simulink model "neoArm_14_05_2024"  (R2023a)
settings: Solver=VariableStepAuto  StartTime=0.0  StopTime=16  FixedStep=0.001  RelTol=1e-3
values from neighbouring files (symbols this model uses):
  dq0 = [0;0;0;0;0]    [neoArm_main.m]
  K = [1000  900]    [neoArm_main.m]
  objectPos = 0.2    [neoArm_main.m]
  orientations = pi/2*[ones(length(temp1),1) zeros(length(temp1),1) zeros(length(temp1),1)]'    [nesneTakip.m]
  q0 = [0;0;0;0;0]    [neoArm_main.m]
  q1 = [pi/2;0;0;0;0]    [neoArm_main.m]
  refPos = 0.0    (= 0)    [neoArm_main.m]
  tDuration = 16    [neoArm_main.m]
  temp3_x = temp3(1,:)    [nokta_duzenle.m]
  temp3_y = temp3(2,:)    [nokta_duzenle.m]
  temp3_z = temp3(3,:)    [nokta_duzenle.m]
  ts = 0.02    [neoArm_main.m]
  tStart = 0.05    [neoArm_main.m]
  waypoints = temp1'    [nesneTakip.m]
  waypointTimes = linspace(0,tDuration,sayi)    [neoArm_main.m]
  weights = [0 0 0 1 1 1]    [neoArm_main.m]
  wp_js_time = [0 0.001 0.002 0.003 0.004 0.005 0.006 0.007 0.008 0.009 0.01 0.011 ... (16001 elements, 16001x1)]    [joint_space_waypoints.mat]    (also in nokta_duzenle.m = wp_joint_space.Time)
undefined symbols (not defined in the file or in its folder): eul2tform, Levenberg, Marquardt, trvec2tform, X, Y, Z
libraries: sm_lib x69, nesl_utility x37, robotcorelib x10, robotmaniplib x9, simulink x2
(part 1 of 3)
settings Model: SimulationMode=accelerator  PacingRate=0.110000  Creator=guven  LastModifiedBy=guven
settings SolverCC: ZeroCrossAlgorithm=Adaptive
settings DataIOCC: ReturnWorkspaceOutputs=off
settings DebuggingCC: IgnoredZcDiagnostic=none
settings ModelReferenceCC: EnableRefExpFcnMdlSchedulingChecks=on

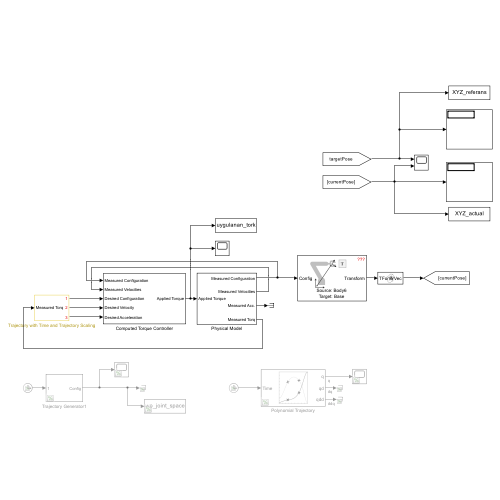
[thumbnail: Simulink's stored preview of the top-level diagram]
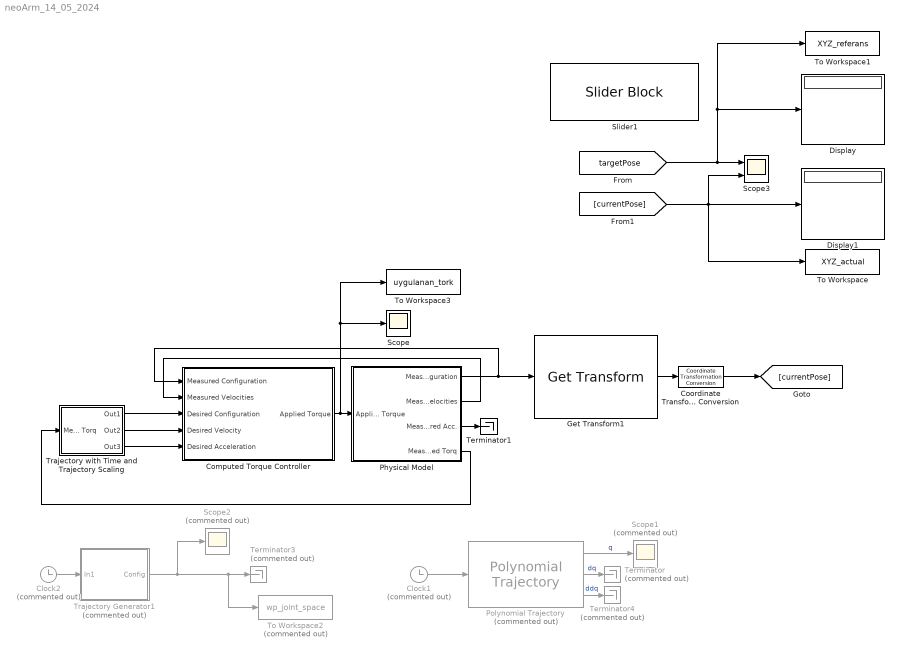
== system neoArm_14_05_2024 ==
  Clock1 : Clock  Commented=on
  Clock2 : Clock  Commented=on
  Computed Torque Controller : Subsystem
  Coordinate Transformation Conversion : robotcorelib/Coordinate Transformation Conversion  InputRepresentation=Homogeneous Transformation  InputEulerSequence=ZYX  ShowTrVecInputPort=on  OutputRepresentation=Translation Vector  OutputEulerSequence=ZYX  ShowTrVecOutputPort=on  SimulateUsing=Interpreted execution
      settings: LibrarySourceBlock=navlib/Utilities/Coordinate Transformation Conversion
  Display : Display
  Display1 : Display
  Get Transform1 : robotmaniplib/Get Transform  RigidBodyTree=neoArm  SourceBody=Body6  TargetBody=Base  SimulateUsing=Interpreted execution
  Physical Model : Subsystem
  Polynomial Trajectory : robotcorelib/Polynomial Trajectory  Commented=on  WaypointSource=Internal  Waypoints=wp_js'  TimePoints=wp_js_time'  TimeInterval=[ 1, 4 ]  Method=Quintic Polynomial  ParameterSource=Internal  VelocityBoundaryCondition=zeros(numel(wp_js_time),5)'  AccelerationBoundaryCondition=zeros(numel(wp_js_time),5)'  SimulateUsing=Interpreted execution
  Scope : Scope
  Scope1 : Scope  Commented=on
  Scope2 : Scope  Commented=on
  Scope3 : Scope  NumInputPorts=2
  Slider1 : SliderBlock  ScaleMin=0.0  ScaleMax=1
  Terminator : Terminator  Commented=on
  Terminator1 : Terminator
  Terminator3 : Terminator  Commented=on
  Terminator4 : Terminator  Commented=on
  To Workspace : ToWorkspace  VariableName=XYZ_actual  SaveFormat=Timeseries  SampleTime=-1
  To Workspace1 : ToWorkspace  VariableName=XYZ_referans  SaveFormat=Timeseries  SampleTime=-1
  To Workspace2 : ToWorkspace  Commented=on  VariableName=wp_joint_space  SaveFormat=Timeseries  SampleTime=-1
  To Workspace3 : ToWorkspace  VariableName=uygulanan_tork  SampleTime=-1
  Trajectory Generator1 : Subsystem  Commented=on
  Trajectory with Time and Trajectory Scaling : Subsystem
  wires:
  Physical Model/2(Measured Velocities) -> Computed Torque Controller/2(Measured Velocities)
  Physical Model/3(Measured Acc.) -> Terminator1/1
  Computed Torque Controller/1(Applied Torque) -> To Workspace3/1, Scope/1, Physical Model/1(Applied Torque)
  [targetPose] -> Display/1, To Workspace1/1, Scope3/1
  [currentPose] -> To Workspace/1, Display1/1, Scope3/2
  Physical Model/4(Measured Torq) -> Trajectory with Time and Trajectory Scaling/1(Measured Torq)
  Trajectory with Time and Trajectory Scaling/1(Out1) -> Computed Torque Controller/3(Desired Configuration)
  Trajectory with Time and Trajectory Scaling/2(Out2) -> Computed Torque Controller/4(Desired Velocity)
  Trajectory with Time and Trajectory Scaling/3(Out3) -> Computed Torque Controller/5(Desired Acceleration)
  Physical Model/1(Measured Configuration) -> Get Transform1/1, Computed Torque Controller/1(Measured Configuration)
  Coordinate Transformation Conversion/1 -> [currentPose]
  Get Transform1/1 -> Coordinate Transformation Conversion/1
  Clock2/1 -> Trajectory Generator1/1(In1)
  Trajectory Generator1/1(Config) -> Scope2/1, To Workspace2/1, Terminator3/1
  Clock1/1 -> Polynomial Trajectory/1
  Polynomial Trajectory/2 -> Terminator/1  "dq"
  Polynomial Trajectory/3 -> Terminator4/1  "ddq"
  Polynomial Trajectory/1 -> Scope1/1  "q"

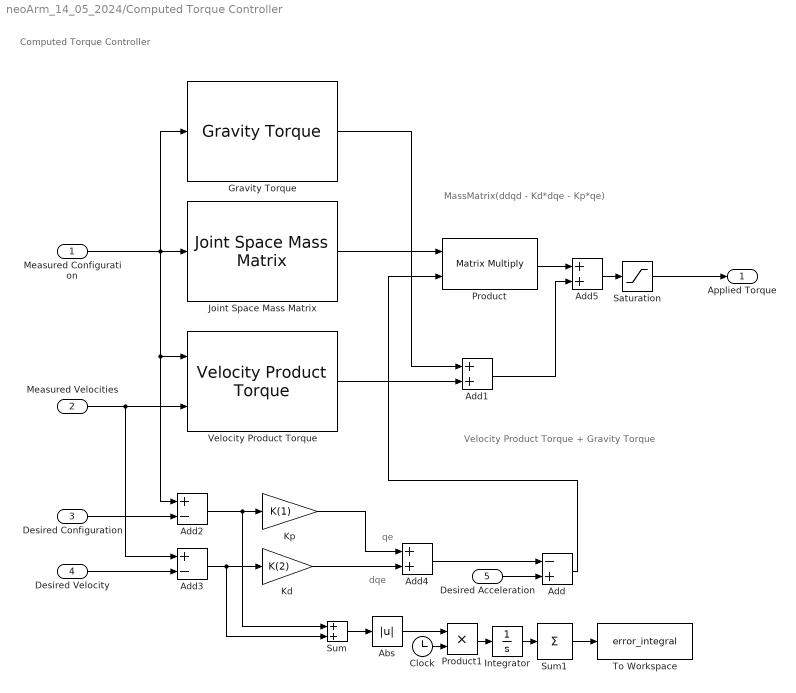
== system neoArm_14_05_2024/Computed Torque Controller ==
  note: Computed Torque Controller
  note: MassMatrix(ddqd - Kd*dqe - Kp*qe)
  note: Velocity Product Torque + Gravity Torque
  note: dqe
  note: qe
  Measured Configuration : Inport
  Measured Velocities : Inport  Port=2
  Desired Configuration : Inport  Port=3
  Desired Velocity : Inport  Port=4
  Desired Acceleration : Inport  Port=5
  Abs : Abs  SaturateOnIntegerOverflow=off
  Add : Sum  Inputs=-+
  Add1 : Sum
  Add2 : Sum  Inputs=+-
  Add3 : Sum  Inputs=+-
  Add4 : Sum
  Add5 : Sum
  Clock : Clock
  Gravity Torque : robotmaniplib/Gravity Torque  RigidBodyTree=neoArm  SimulateUsing=Interpreted execution
  Integrator : Integrator
  Joint Space Mass Matrix : robotmaniplib/Joint Space Mass Matrix  RigidBodyTree=neoArm  SimulateUsing=Interpreted execution
  Kd : Gain  Gain=K(2)
  Kp : Gain  Gain=K(1)
  Product : Product  Multiplication=Matrix(*)
  Product1 : Product
  Saturation : Saturate  UpperLimit=100  LowerLimit=-100
  Sum : Sum
  Sum1 : Sum  Inputs=+
  To Workspace : ToWorkspace  VariableName=error_integral  SampleTime=-1
      settings: Save2DSignal=2-D array (concatenate along first dimension)
  Velocity Product Torque : robotmaniplib/Velocity Product Torque  RigidBodyTree=neoArm  SimulateUsing=Interpreted execution
  Applied Torque : Outport  VectorParamsAs1DForOutWhenUnconnected=off
  wires:
  Add5/1 -> Saturation/1
  Velocity Product Torque/1 -> Add1/2
  Gravity Torque/1 -> Add1/1
  Add1/1 -> Add5/2
  Product/1 -> Add5/1
  Kd/1 -> Add4/2
  Kp/1 -> Add4/1
  Add3/1 -> Sum/2, Kd/1
  Add2/1 -> Sum/1, Kp/1
  Desired Configuration/1 -> Add2/2
  Add/1 -> Product/2
  Desired Acceleration/1 -> Add/2
  Add4/1 -> Add/1
  Measured Velocities/1 -> Velocity Product Torque/2, Add3/1
  Measured Configuration/1 -> Gravity Torque/1, Add2/1, Velocity Product Torque/1, Joint Space Mass Matrix/1
  Joint Space Mass Matrix/1 -> Product/1
  Desired Velocity/1 -> Add3/2
  Sum/1 -> Abs/1
  Clock/1 -> Product1/2
  Abs/1 -> Product1/1
  Product1/1 -> Integrator/1
  Integrator/1 -> Sum1/1
  Sum1/1 -> To Workspace/1
  Saturation/1 -> Applied Torque/1

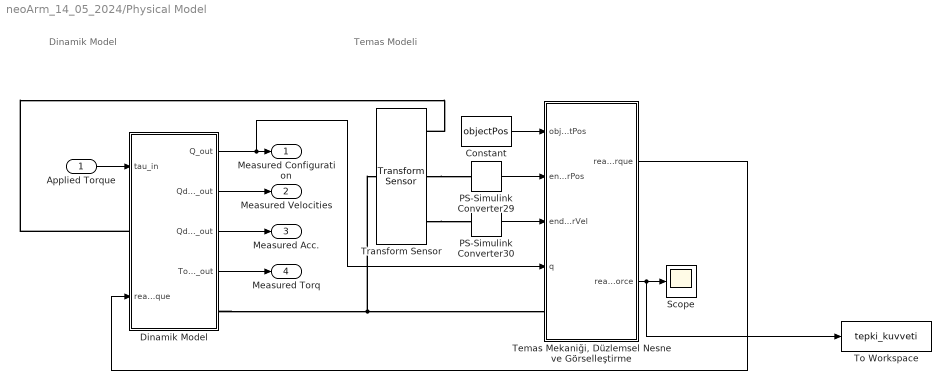
== system neoArm_14_05_2024/Physical Model ==
  note: Temas Modeli
  note: Dinamik Model
  Applied Torque : Inport
  Constant : Constant  Value=objectPos
  Dinamik Model : Subsystem
      settings: PortSchema="{\"entries\":[{\"content\":{\"sides\":[{\"content\":{\"connectorIds\":[\"In1\",\"LConn1\",\"In2\"]},\"type\":\"ConnectorPlacement.EquallySpacedRectSide\",\"uuid\":\"664d0935-1bf3-446c-8732-22792c17880e\"},{\"content\":{\"connectorIds\":[\"Out1\",\"Out2\",\"Out3\",\"Out4\",\"RConn1\"],\"side\":\"RIGHT\"},\"type\":\"ConnectorPlacement.EquallySpacedRectSide\",\"uuid\":\"708aa5df-690c-4635-a2be-b9b7c80f1d52\"},{\"content\":{\"side\":\"TOP\"},\"type\":\"ConnectorPlacement.EquallySpacedRectSide\",\"uuid\":\"c49793cc-4428-4e38-a5f9-d7e5674b8e19\"}]},\"type\":\"ConnectorPlacement.EquallySpacedConnector\",\"uuid\":\"e38b11a5-9e9e-43e5-b16b-ed3f208c0f6a\"}],\"packageUris\":[\"http://schema.mathworks.com/mf0/Connector/R2020b\"],\"version\":\"1.0\"}"
  PS-Simulink Converter29 : nesl_utility/PS-Simulink Converter  PhysicalDomain=network_engine_domain  SubClassName=ps_output  LeftPortType=input  RightPortType=output  PseudoPeriodic=off  Frequencies=[]  VectorFormat=1-D array  Unit=1  AffineConversion=off
  PS-Simulink Converter30 : nesl_utility/PS-Simulink Converter  PhysicalDomain=network_engine_domain  SubClassName=ps_output  LeftPortType=input  RightPortType=output  PseudoPeriodic=off  Frequencies=[]  VectorFormat=1-D array  Unit=1  AffineConversion=off
  Scope : Scope
  "Temas Mekaniği, Düzlemsel Nesne ve Görselleştirme" : Subsystem
  To Workspace : ToWorkspace  VariableName=tepki_kuvveti  SampleTime=-1
  Transform Sensor : sm_lib/Frames and Transforms/Transform Sensor  MeasurementFrame=World  RotationSequence=XYX  SenseAngle=off  SenseAxis=off  SenseQ=off  SenseR=off  SenseRotationSequence=off  SenseOmegaX=off  SenseOmegaY=off  SenseOmegaZ=off  SenseQDot=off  SenseRDot=off  SenseRotationSequenceDot=off  SenseAlphaX=off  SenseAlphaY=off  SenseAlphaZ=off  SenseQDDot=off  SenseRDDot=off  SenseX=on  SenseY=off  SenseZ=off  SenseRad=off  SenseAzim=off  SenseDist=off  SenseInc=off  SenseXDot=on  SenseYDot=off  SenseZDot=off  SenseRadDot=off  SenseAzimDot=off  SenseDistDot=off  SenseIncDot=off  SenseXDDot=off  SenseYDDot=off  SenseZDDot=off  SenseRadDDot=off  SenseAzimDDot=off  SenseDistDDot=off  SenseIncDDot=off
  Measured Configuration : Outport
  Measured Velocities : Outport  Port=2
  Measured Acc. : Outport  Port=3
  Measured Torq : Outport  Port=4
  wires:
  "Temas Mekaniği, Düzlemsel Nesne ve Görselleştirme"/2(reaction force) -> To Workspace/1, Scope/1
  PS-Simulink Converter29/1 -> "Temas Mekaniği, Düzlemsel Nesne ve Görselleştirme"/2(endeffectorPos)
  PS-Simulink Converter30/1 -> "Temas Mekaniği, Düzlemsel Nesne ve Görselleştirme"/3(endeffectorVel)
  "Temas Mekaniği, Düzlemsel Nesne ve Görselleştirme"/1(reaction torque) -> Dinamik Model/2(reaction torque)
  Constant/1 -> "Temas Mekaniği, Düzlemsel Nesne ve Görselleştirme"/1(objectPos)
  Dinamik Model/1(Q_out) -> Measured Configuration/1, "Temas Mekaniği, Düzlemsel Nesne ve Görselleştirme"/4(q)
  Dinamik Model/2(Qdot_out) -> Measured Velocities/1
  Dinamik Model/3(Qddot_out) -> Measured Acc./1
  Dinamik Model/4(Torq_out) -> Measured Torq/1
  Applied Torque/1 -> Dinamik Model/1(tau_in)
  connections:
  Transform Sensor/RConn3 -- PS-Simulink Converter30/LConn1
  Transform Sensor/RConn2 -- PS-Simulink Converter29/LConn1
  Dinamik Model/RConn1 -- "Temas Mekaniği, Düzlemsel Nesne ve Görselleştirme"/LConn1 -- Transform Sensor/LConn1
  Dinamik Model/LConn1 -- Transform Sensor/RConn1

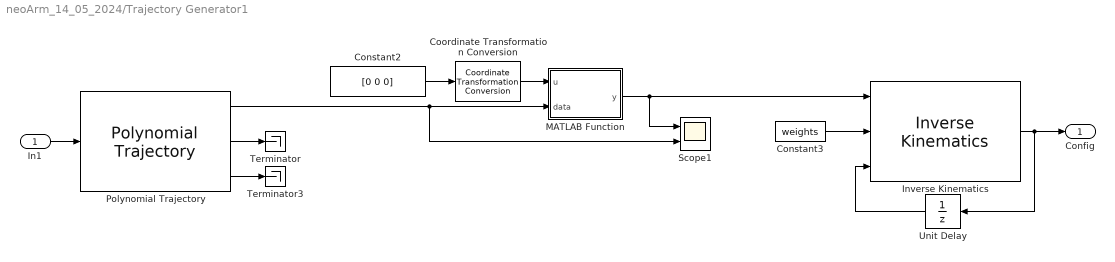
== system neoArm_14_05_2024/Trajectory Generator1 ==
  In1 : Inport
  Constant2 : Constant  Value=[0 0 0]
  Constant3 : Constant  Value=weights  VectorParams1D=off
  Coordinate Transformation Conversion : robotcorelib/Coordinate Transformation Conversion  InputRepresentation=Euler Angles  InputEulerSequence=ZYX  ShowTrVecInputPort=off  OutputRepresentation=Homogeneous Transformation  OutputEulerSequence=ZYX  ShowTrVecOutputPort=on  SimulateUsing=Interpreted execution
      settings: LibrarySourceBlock=navlib/Utilities/Coordinate Transformation Conversion
  Inverse Kinematics : robotmaniplib/Inverse Kinematics  RigidBodyTree=neoArm  EndEffector=Body6  ShowInfo=off  SolverName=BFGS Gradient Projection  EnforceJointLimits=on  MaxIterations=1500  MaxTime=10  GradientTolerance=1e-7  SolutionTolerance=1e-6  StepTolerance=1e-14  ErrorChangeTolerance=1e-12  UseErrorDamping=on  DampingBias=0.0025  SimulateUsing=Interpreted execution
  MATLAB Function : MATLAB Function  TreatAsAtomicUnit=on
  Polynomial Trajectory : robotcorelib/Polynomial Trajectory  WaypointSource=Internal  Waypoints=[temp3_x; temp3_y; temp3_z]  TimePoints=waypointTimes  TimeInterval=[ 1, 4 ]  Method=Cubic Polynomial  ParameterSource=Internal  VelocityBoundaryCondition=zeros( numel(waypointTimes),3 )'  AccelerationBoundaryCondition=zeros( 2, 5 )  SimulateUsing=Interpreted execution
  Scope1 : Scope  NumInputPorts=2
  Terminator : Terminator
  Terminator3 : Terminator
  Unit Delay : UnitDelay  InitialCondition=q0  SampleTime=-1  HasFrameUpgradeWarning=on
  Config : Outport
  wires:
  Inverse Kinematics/1 -> Config/1, Unit Delay/1
  Polynomial Trajectory/1 -> Scope1/2, MATLAB Function/2(data)
  Constant2/1 -> Coordinate Transformation Conversion/1
  MATLAB Function/1(y) -> Scope1/1, Inverse Kinematics/1
  Unit Delay/1 -> Inverse Kinematics/3
  Constant3/1 -> Inverse Kinematics/2
  Coordinate Transformation Conversion/1 -> MATLAB Function/1(u)
  In1/1 -> Polynomial Trajectory/1
  Polynomial Trajectory/2 -> Terminator/1
  Polynomial Trajectory/3 -> Terminator3/1

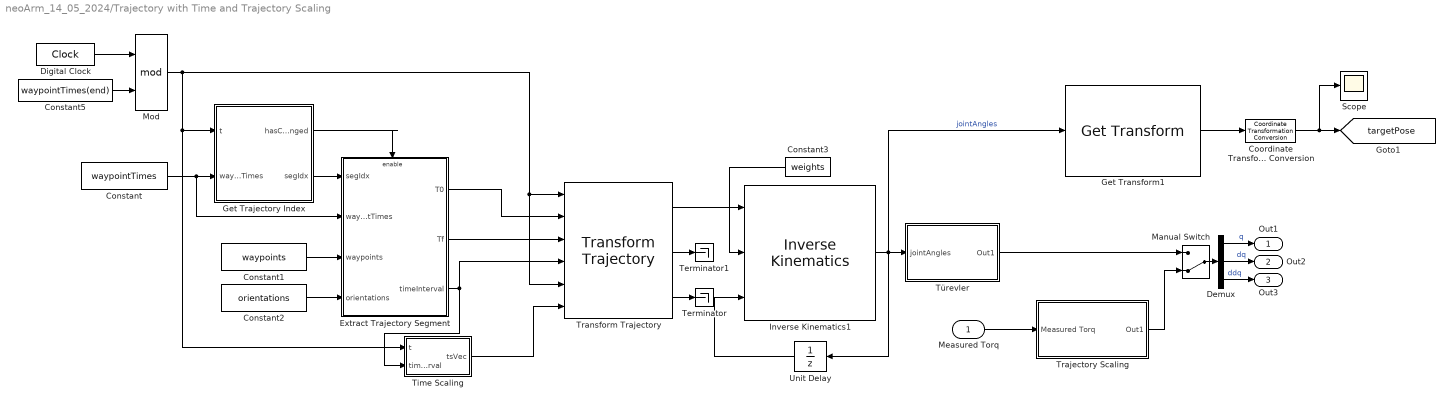
== system neoArm_14_05_2024/Trajectory with Time and Trajectory Scaling ==
  Measured Torq : Inport
  Constant : Constant  Value=waypointTimes
  Constant1 : Constant  Value=waypoints
  Constant2 : Constant  Value=orientations
  Constant3 : Constant  Value=weights  VectorParams1D=off
  Constant5 : Constant  Value=waypointTimes(end)
  Coordinate Transformation Conversion : robotcorelib/Coordinate Transformation Conversion  InputRepresentation=Homogeneous Transformation  InputEulerSequence=ZYX  ShowTrVecInputPort=on  OutputRepresentation=Translation Vector  OutputEulerSequence=ZYX  ShowTrVecOutputPort=on  SimulateUsing=Interpreted execution
      settings: LibrarySourceBlock=navlib/Utilities/Coordinate Transformation Conversion
  Demux : Demux  Outputs=3
  Digital Clock : DigitalClock  SampleTime=ts
  Extract Trajectory Segment : Subsystem
  Get Trajectory Index : MATLAB Function  TreatAsAtomicUnit=on
  Get Transform1 : robotmaniplib/Get Transform  RigidBodyTree=neoArm  SourceBody=Body6  TargetBody=Base  SimulateUsing=Interpreted execution
  Inverse Kinematics1 : robotmaniplib/Inverse Kinematics  RigidBodyTree=neoArm  EndEffector=Body6  ShowInfo=off  SolverName=Levenberg-Marquardt  EnforceJointLimits=on  MaxIterations=1500  MaxTime=10  GradientTolerance=1e-7  SolutionTolerance=1e-6  StepTolerance=1e-14  ErrorChangeTolerance=1e-12  UseErrorDamping=on  DampingBias=0.0025  SimulateUsing=Interpreted execution
  Manual Switch : ManualSwitch  CurrentSetting=0
  Mod : Math  Operator=mod  SignedPower=on
  Scope : Scope
  Terminator : Terminator
  Terminator1 : Terminator
  Time Scaling : Subsystem
  Trajectory Scaling : Subsystem
  Transform Trajectory : robotcorelib/Transform Trajectory  WaypointSource=External  T0=trvec2tform( [ 1, 10, -1 ] )  TF=eul2tform( [ 0, pi, pi / 2 ] )  TimeInterval=[ 2, 3 ]  CustomTimeScaling=on  ParameterSource=External  TSTime=2:0.1:3  TimeScaling=[ 0:0.1:1; ones( 1, 11 ); zeros( 1, 11 ) ]  SimulateUsing=Interpreted execution
  Türevler : Subsystem
  Unit Delay : UnitDelay  InitialCondition=q0  SampleTime=-1  HasFrameUpgradeWarning=on
  Out1 : Outport
  Out2 : Outport  Port=2
  Out3 : Outport  Port=3
  tag scope: targetPose=global
  wires:
  Extract Trajectory Segment/2(Tf) -> Transform Trajectory/3
  Get Trajectory Index/2(segIdx) -> Extract Trajectory Segment/1(segIdx)
  Constant5/1 -> Mod/2
  Constant2/1 -> Extract Trajectory Segment/4(orientations)
  Unit Delay/1 -> Inverse Kinematics1/3
  Transform Trajectory/1 -> Inverse Kinematics1/1
  Mod/1 -> Get Trajectory Index/1(t), Time Scaling/1(t), Transform Trajectory/5, Transform Trajectory/1
  Extract Trajectory Segment/3(timeInterval) -> Time Scaling/2(timeInterval), Transform Trajectory/4
  Constant/1 -> Extract Trajectory Segment/2(waypointTimes), Get Trajectory Index/2(waypointTimes)
  Constant1/1 -> Extract Trajectory Segment/3(waypoints)
  Get Trajectory Index/1(hasChanged) -> Extract Trajectory Segment/Enable
  Constant3/1 -> Inverse Kinematics1/2
  Extract Trajectory Segment/1(T0) -> Transform Trajectory/2
  Transform Trajectory/3 -> Terminator/1
  Transform Trajectory/2 -> Terminator1/1
  Demux/3 -> Out3/1  "ddq"
  Demux/1 -> Out1/1  "q"
  Demux/2 -> Out2/1  "dq"
  Coordinate Transformation Conversion/1 -> Scope/1, [targetPose]
  Get Transform1/1 -> Coordinate Transformation Conversion/1
  Inverse Kinematics1/1 -> Unit Delay/1, Get Transform1/1, Türevler/1(jointAngles)  "jointAngles"
  Time Scaling/1(tsVec) -> Transform Trajectory/6
  Digital Clock/1 -> Mod/1
  Türevler/1(Out1) -> Manual Switch/1
  Manual Switch/1 -> Demux/1
  Measured Torq/1 -> Trajectory Scaling/1(Measured Torq)
  Trajectory Scaling/1(Out1) -> Manual Switch/2

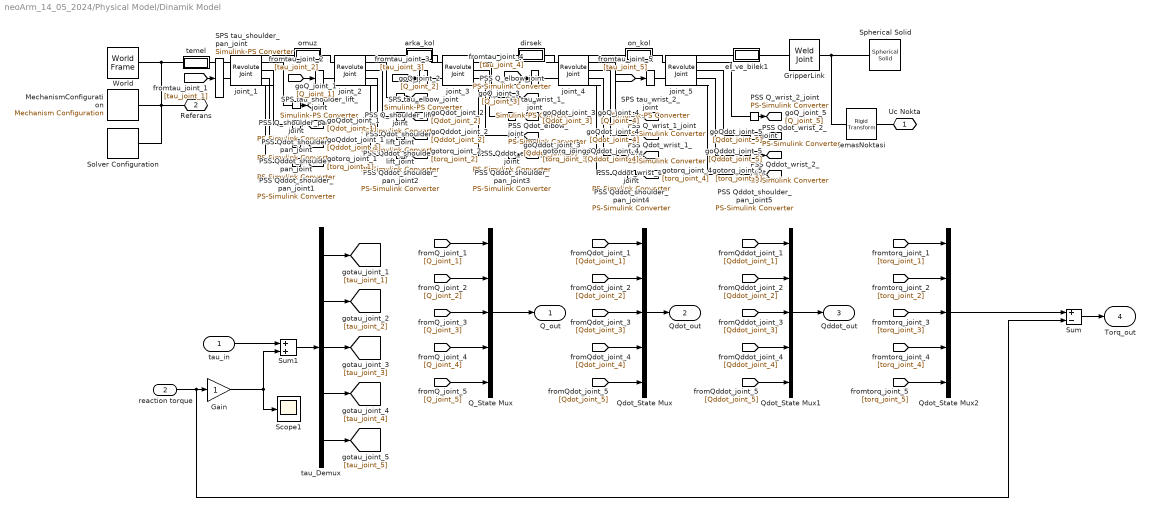
== system neoArm_14_05_2024/Physical Model/Dinamik Model ==
  tau_in : Inport
  reaction torque : Inport  Port=2
  Gain : Gain
  GripperLink : sm_lib/Joints/Weld Joint  JointMode=Normal  SenseConstraintForce=off  SenseConstraintForceX=off  SenseConstraintForceY=off  SenseConstraintForceZ=off  SenseConstraintTorque=off  SenseConstraintTorqueX=off  SenseConstraintTorqueY=off  SenseConstraintTorqueZ=off  SenseTotalForce=off  SenseTotalForceX=off  SenseTotalForceY=off  SenseTotalForceZ=off  SenseTotalTorque=off  SenseTotalTorqueX=off  SenseTotalTorqueY=off  SenseTotalTorqueZ=off  CompositeWrenchDir=BaseOnFollower  CompositeWrenchFrame=BaseFrame
  MechanismConfiguration : sm_lib/Utilities/Mechanism Configuration  UniformGravity=Constant  GravityVector=[0, 0, -9.80655]  GravityVectorUnits=m/s^2  LinearizationDelta=0.001  JointModeTransitionNonlinearIterations=2
  PSS Q_elbow_joint : nesl_utility/PS-Simulink Converter  PhysicalDomain=network_engine_domain  SubClassName=ps_output  LeftPortType=input  RightPortType=output  PseudoPeriodic=off  Frequencies=[]  VectorFormat=inherit  Unit=inherit  AffineConversion=off
  PSS Q_shoulder_lift_joint : nesl_utility/PS-Simulink Converter  PhysicalDomain=network_engine_domain  SubClassName=ps_output  LeftPortType=input  RightPortType=output  PseudoPeriodic=off  Frequencies=[]  VectorFormat=inherit  Unit=inherit  AffineConversion=off
  PSS Q_shoulder_pan_joint : nesl_utility/PS-Simulink Converter  PhysicalDomain=network_engine_domain  SubClassName=ps_output  LeftPortType=input  RightPortType=output  PseudoPeriodic=off  Frequencies=[]  VectorFormat=inherit  Unit=inherit  AffineConversion=off
  PSS Q_wrist_1_joint : nesl_utility/PS-Simulink Converter  PhysicalDomain=network_engine_domain  SubClassName=ps_output  LeftPortType=input  RightPortType=output  PseudoPeriodic=off  Frequencies=[]  VectorFormat=inherit  Unit=inherit  AffineConversion=off
  PSS Q_wrist_2_joint : nesl_utility/PS-Simulink Converter  PhysicalDomain=network_engine_domain  SubClassName=ps_output  LeftPortType=input  RightPortType=output  PseudoPeriodic=off  Frequencies=[]  VectorFormat=inherit  Unit=inherit  AffineConversion=off
  PSS Qddot_elbow_joint : nesl_utility/PS-Simulink Converter  PhysicalDomain=network_engine_domain  SubClassName=ps_output  LeftPortType=input  RightPortType=output  PseudoPeriodic=off  Frequencies=[]  VectorFormat=inherit  Unit=inherit  AffineConversion=off
  PSS Qddot_shoulder_lift_joint : nesl_utility/PS-Simulink Converter  PhysicalDomain=network_engine_domain  SubClassName=ps_output  LeftPortType=input  RightPortType=output  PseudoPeriodic=off  Frequencies=[]  VectorFormat=inherit  Unit=inherit  AffineConversion=off
  PSS Qddot_shoulder_pan_joint{,1..5} (6 alike) : nesl_utility/PS-Simulink Converter  PhysicalDomain=network_engine_domain  SubClassName=ps_output  LeftPortType=input  RightPortType=output  PseudoPeriodic=off  Frequencies=[]  VectorFormat=inherit  Unit=inherit  AffineConversion=off
  PSS Qddot_wrist_1_joint : nesl_utility/PS-Simulink Converter  PhysicalDomain=network_engine_domain  SubClassName=ps_output  LeftPortType=input  RightPortType=output  PseudoPeriodic=off  Frequencies=[]  VectorFormat=inherit  Unit=inherit  AffineConversion=off
  PSS Qddot_wrist_2_joint : nesl_utility/PS-Simulink Converter  PhysicalDomain=network_engine_domain  SubClassName=ps_output  LeftPortType=input  RightPortType=output  PseudoPeriodic=off  Frequencies=[]  VectorFormat=inherit  Unit=inherit  AffineConversion=off
  PSS Qdot_elbow_joint : nesl_utility/PS-Simulink Converter  PhysicalDomain=network_engine_domain  SubClassName=ps_output  LeftPortType=input  RightPortType=output  PseudoPeriodic=off  Frequencies=[]  VectorFormat=inherit  Unit=inherit  AffineConversion=off
  PSS Qdot_shoulder_lift_joint : nesl_utility/PS-Simulink Converter  PhysicalDomain=network_engine_domain  SubClassName=ps_output  LeftPortType=input  RightPortType=output  PseudoPeriodic=off  Frequencies=[]  VectorFormat=inherit  Unit=inherit  AffineConversion=off
  PSS Qdot_shoulder_pan_joint : nesl_utility/PS-Simulink Converter  PhysicalDomain=network_engine_domain  SubClassName=ps_output  LeftPortType=input  RightPortType=output  PseudoPeriodic=off  Frequencies=[]  VectorFormat=inherit  Unit=inherit  AffineConversion=off
  PSS Qdot_wrist_1_joint : nesl_utility/PS-Simulink Converter  PhysicalDomain=network_engine_domain  SubClassName=ps_output  LeftPortType=input  RightPortType=output  PseudoPeriodic=off  Frequencies=[]  VectorFormat=inherit  Unit=inherit  AffineConversion=off
  PSS Qdot_wrist_2_joint : nesl_utility/PS-Simulink Converter  PhysicalDomain=network_engine_domain  SubClassName=ps_output  LeftPortType=input  RightPortType=output  PseudoPeriodic=off  Frequencies=[]  VectorFormat=inherit  Unit=inherit  AffineConversion=off
  Q_State Mux : Mux  Inputs=5
  Qdot_State Mux : Mux  Inputs=5
  Qdot_State Mux1 : Mux  Inputs=5
  Qdot_State Mux2 : Mux  Inputs=5
  SPS tau_elbow_joint : nesl_utility/Simulink-PS Converter  PhysicalDomain=network_engine_domain  SubClassName=ps_input  LeftPortType=input  RightPortType=output  PseudoPeriodic=off  Frequencies=[]  NoiseDistribution=none  NoiseParameters=[]  Unit=1  AffineConversion=off  FilteringAndDerivatives=filter  SimscapeFilterOrder=2  InputFilterTimeConstant=0.001  UdotUserProvided=0
  SPS tau_shoulder_lift_joint : nesl_utility/Simulink-PS Converter  PhysicalDomain=network_engine_domain  SubClassName=ps_input  LeftPortType=input  RightPortType=output  PseudoPeriodic=off  Frequencies=[]  NoiseDistribution=none  NoiseParameters=[]  Unit=1  AffineConversion=off  FilteringAndDerivatives=filter  SimscapeFilterOrder=2  InputFilterTimeConstant=0.001  UdotUserProvided=0
  SPS tau_shoulder_pan_joint : nesl_utility/Simulink-PS Converter  PhysicalDomain=network_engine_domain  SubClassName=ps_input  LeftPortType=input  RightPortType=output  PseudoPeriodic=off  Frequencies=[]  NoiseDistribution=none  NoiseParameters=[]  Unit=1  AffineConversion=off  FilteringAndDerivatives=filter  SimscapeFilterOrder=2  InputFilterTimeConstant=0.001  UdotUserProvided=0
  SPS tau_wrist_1_joint : nesl_utility/Simulink-PS Converter  PhysicalDomain=network_engine_domain  SubClassName=ps_input  LeftPortType=input  RightPortType=output  PseudoPeriodic=off  Frequencies=[]  NoiseDistribution=none  NoiseParameters=[]  Unit=1  AffineConversion=off  FilteringAndDerivatives=filter  SimscapeFilterOrder=2  InputFilterTimeConstant=0.001  UdotUserProvided=0
  SPS tau_wrist_2_joint : nesl_utility/Simulink-PS Converter  PhysicalDomain=network_engine_domain  SubClassName=ps_input  LeftPortType=input  RightPortType=output  PseudoPeriodic=off  Frequencies=[]  NoiseDistribution=none  NoiseParameters=[]  Unit=1  AffineConversion=off  FilteringAndDerivatives=filter  SimscapeFilterOrder=2  InputFilterTimeConstant=0.001  UdotUserProvided=0
  Scope1 : Scope
  Solver Configuration : nesl_utility/Solver Configuration  PhysicalDomain=network_engine_domain  SubClassName=solver  LeftPortType=input  RightPortType=generic  Tones=[]  Harmonics=[]  SimulateNoise=off  Profile=off  UseLocalSampling=off  EnableSwitchedLinearOptims=on  FrequencyDomain=off  UseCCode=off  RelTol=0.001  AbsTol=0.001  MinStep=1e-09  ToWorkspace=off  RevertToSquareIcSolve=off  NumHomotopyIterations=100  PhasorMode=off  PhasorModeNumHarmonics=1  ConsistencySolver=NEWTON_XTOL_AFTER_FTOL  IndexReductionMethod=DerivativeReplacement  DoDC=off  ResidualTolerance=1e-09  ConsistencyTolSource=GLOBAL  ConsistencyAbsTol=0.001  ConsistencyRelTol=0.001  ConsistencyTolFactor=1e-9  UseLocalSolver=off  LocalSolverChoice=NE_BACKWARD_EULER_ADVANCER  ResolveIndetEquations=on  FunctionEvalNumThread=1  LocalSolverSampleTime=0.001  DoFixedCost=off  MaxNonlinIter=3  MaxModeIter=2  ComputeImpulses=off  ImpulseIterations=2  LinearAlgebra=auto  LinearAlgebraNumThread=0  EquationFormulation=NE_TIME_EF  DelaysMemoryBudget=1024  AutomaticFiltering=on  FilteringTimeConstant=0.001  PartitionStorageMethod=AS_NEEDED  PartitionMemoryBudget=1024  PartitionMethod=ROBUST
  Spherical Solid : sm_lib/Body Elements/Spherical Solid  GraphicAmbientColor=[0.15 0.15 0.15 1.0]  BasedOnType=Density  CenterOfMass=[0 0 0]  CenterOfMassUnits=m  GraphicDiffuseColor=[0.5 0.5 0.5]  Density=100  DensityUnits=kg/m^3  DoExposeReferenceFrame=on  GraphicEmissiveColor=[0.0 0.0 0.0 1.0]  ExportEntireGeometry=off  SerializedExposedGeometries=<ExposedGeometries/>  SerializedFrames=<Frames/>  MarkerShape=Sphere  MarkerSize=10  GraphicType=FromGeometry  InertiaType=CalculateFromGeometry  Mass=1  MassUnits=kg  MomentsOfInertia=[1 1 1]  MomentsOfInertiaUnits=kg*m^2  GraphicOpacity=1.0  ProductsOfInertia=[0 0 0]  ProductsOfInertiaUnits=kg*m^2  GraphicShininess=75  GraphicSpecularColor=[0.5 0.5 0.5 1.0]  SphereRadius=0.045  SphereRadiusUnits=m  GraphicVisPropType=SimpleVisualProperties
  Sum : Sum  Inputs=+-
  Sum1 : Sum
  World : sm_lib/Frames and Transforms/World Frame
  arka_kol : Subsystem
  dirsek : Subsystem
  el_ve_bilek1 : Subsystem
  joint_1 : sm_lib/Joints/Revolute Joint  JointMode=Normal  SenseConstraintForce=off  SenseConstraintForceX=off  SenseConstraintForceY=off  SenseConstraintForceZ=off  SenseConstraintTorque=off  SenseConstraintTorqueX=off  SenseConstraintTorqueY=off  SenseConstraintTorqueZ=off  SenseTotalForce=off  SenseTotalForceX=off  SenseTotalForceY=off  SenseTotalForceZ=off  SenseTotalTorque=off  SenseTotalTorqueX=off  SenseTotalTorqueY=off  SenseTotalTorqueZ=off  CompositeWrenchDir=FollowerOnBase  CompositeWrenchFrame=BaseFrame  EquilibriumPosition=0  EquilibriumPositionUnits=deg  SpringStiffness=0  SpringStiffnessUnits=N*m/deg  DampingCoefficient=0  DampingCoefficientUnits=kg*m^2/(rad*s)  TorqueActuationMode=InputTorque  MotionActuationMode=ComputedMotion  SensePosition=on  SenseVelocity=on  SenseAcceleration=on  SenseTorqueForce=on  SenseLowerLimitTorqueForce=off  SenseUpperLimitTorqueForce=off  LowerLimitSpecify=off  LowerLimitBound=-180  LowerLimitBoundUnits=deg  LowerLimitStiffness=0  LowerLimitStiffnessUnits=N*m/deg  LowerLimitDamping=0  LowerLimitDampingUnits=N*m/(deg/s)  LowerLimitTransitionRegionWidth=0.1  LowerLimitTransitionRegionWidthUnits=deg  UpperLimitSpecify=off  UpperLimitBound=180  UpperLimitBoundUnits=rad  UpperLimitStiffness=0  UpperLimitStiffnessUnits=N*m/deg  UpperLimitDamping=0  UpperLimitDampingUnits=N*m/(deg/s)  UpperLimitTransitionRegionWidth=0.1  UpperLimitTransitionRegionWidthUnits=deg  PositionTargetSpecify=on  PositionTargetPriority=High  PositionTargetValue=q0(1)  PositionTargetValueUnits=rad  VelocityTargetSpecify=on  VelocityTargetPriority=High  VelocityTargetValue=dq0(1)  VelocityTargetValueUnits=rad/s
  joint_2 : sm_lib/Joints/Revolute Joint  JointMode=Normal  SenseConstraintForce=off  SenseConstraintForceX=off  SenseConstraintForceY=off  SenseConstraintForceZ=off  SenseConstraintTorque=off  SenseConstraintTorqueX=off  SenseConstraintTorqueY=off  SenseConstraintTorqueZ=off  SenseTotalForce=off  SenseTotalForceX=off  SenseTotalForceY=off  SenseTotalForceZ=off  SenseTotalTorque=off  SenseTotalTorqueX=off  SenseTotalTorqueY=off  SenseTotalTorqueZ=off  CompositeWrenchDir=FollowerOnBase  CompositeWrenchFrame=BaseFrame  EquilibriumPosition=0  EquilibriumPositionUnits=deg  SpringStiffness=0  SpringStiffnessUnits=N*m/deg  DampingCoefficient=0  DampingCoefficientUnits=kg*m^2/(rad*s)  TorqueActuationMode=InputTorque  MotionActuationMode=ComputedMotion  SensePosition=on  SenseVelocity=on  SenseAcceleration=on  SenseTorqueForce=on  SenseLowerLimitTorqueForce=off  SenseUpperLimitTorqueForce=off  LowerLimitSpecify=off  LowerLimitBound=-pi/2  LowerLimitBoundUnits=rad  LowerLimitStiffness=0  LowerLimitStiffnessUnits=N*m/deg  LowerLimitDamping=0  LowerLimitDampingUnits=N*m/(deg/s)  LowerLimitTransitionRegionWidth=0.1  LowerLimitTransitionRegionWidthUnits=deg  UpperLimitSpecify=off  UpperLimitBound=pi/2  UpperLimitBoundUnits=rad  UpperLimitStiffness=0  UpperLimitStiffnessUnits=N*m/deg  UpperLimitDamping=0  UpperLimitDampingUnits=N*m/(deg/s)  UpperLimitTransitionRegionWidth=0.1  UpperLimitTransitionRegionWidthUnits=deg  PositionTargetSpecify=on  PositionTargetPriority=High  PositionTargetValue=q0(2)  PositionTargetValueUnits=rad  VelocityTargetSpecify=on  VelocityTargetPriority=High  VelocityTargetValue=dq0(2)  VelocityTargetValueUnits=rad/s
  joint_3 : sm_lib/Joints/Revolute Joint  JointMode=Normal  SenseConstraintForce=off  SenseConstraintForceX=off  SenseConstraintForceY=off  SenseConstraintForceZ=off  SenseConstraintTorque=off  SenseConstraintTorqueX=off  SenseConstraintTorqueY=off  SenseConstraintTorqueZ=off  SenseTotalForce=off  SenseTotalForceX=off  SenseTotalForceY=off  SenseTotalForceZ=off  SenseTotalTorque=off  SenseTotalTorqueX=off  SenseTotalTorqueY=off  SenseTotalTorqueZ=off  CompositeWrenchDir=FollowerOnBase  CompositeWrenchFrame=BaseFrame  EquilibriumPosition=0  EquilibriumPositionUnits=deg  SpringStiffness=0  SpringStiffnessUnits=N*m/deg  DampingCoefficient=0  DampingCoefficientUnits=kg*m^2/(rad*s)  TorqueActuationMode=InputTorque  MotionActuationMode=ComputedMotion  SensePosition=on  SenseVelocity=on  SenseAcceleration=on  SenseTorqueForce=on  SenseLowerLimitTorqueForce=off  SenseUpperLimitTorqueForce=off  LowerLimitSpecify=off  LowerLimitBound=-pi/2  LowerLimitBoundUnits=rad  LowerLimitStiffness=0  LowerLimitStiffnessUnits=N*m/deg  LowerLimitDamping=0  LowerLimitDampingUnits=N*m/(deg/s)  LowerLimitTransitionRegionWidth=0.1  LowerLimitTransitionRegionWidthUnits=deg  UpperLimitSpecify=off  UpperLimitBound=pi/2  UpperLimitBoundUnits=rad  UpperLimitStiffness=0  UpperLimitStiffnessUnits=N*m/deg  UpperLimitDamping=0  UpperLimitDampingUnits=N*m/(deg/s)  UpperLimitTransitionRegionWidth=0.1  UpperLimitTransitionRegionWidthUnits=deg  PositionTargetSpecify=on  PositionTargetPriority=High  PositionTargetValue=q0(3)  PositionTargetValueUnits=rad  VelocityTargetSpecify=on  VelocityTargetPriority=High  VelocityTargetValue=dq0(3)  VelocityTargetValueUnits=rad/s
  joint_4 : sm_lib/Joints/Revolute Joint  JointMode=Normal  SenseConstraintForce=off  SenseConstraintForceX=off  SenseConstraintForceY=off  SenseConstraintForceZ=off  SenseConstraintTorque=off  SenseConstraintTorqueX=off  SenseConstraintTorqueY=off  SenseConstraintTorqueZ=off  SenseTotalForce=off  SenseTotalForceX=off  SenseTotalForceY=off  SenseTotalForceZ=off  SenseTotalTorque=off  SenseTotalTorqueX=off  SenseTotalTorqueY=off  SenseTotalTorqueZ=off  CompositeWrenchDir=FollowerOnBase  CompositeWrenchFrame=BaseFrame  EquilibriumPosition=0  EquilibriumPositionUnits=deg  SpringStiffness=0  SpringStiffnessUnits=N*m/deg  DampingCoefficient=0  DampingCoefficientUnits=kg*m^2/(rad*s)  TorqueActuationMode=InputTorque  MotionActuationMode=ComputedMotion  SensePosition=on  SenseVelocity=on  SenseAcceleration=on  SenseTorqueForce=on  SenseLowerLimitTorqueForce=off  SenseUpperLimitTorqueForce=off  LowerLimitSpecify=off  LowerLimitBound=-pi/2  LowerLimitBoundUnits=rad  LowerLimitStiffness=0  LowerLimitStiffnessUnits=N*m/deg  LowerLimitDamping=0  LowerLimitDampingUnits=N*m/(deg/s)  LowerLimitTransitionRegionWidth=0.1  LowerLimitTransitionRegionWidthUnits=deg  UpperLimitSpecify=off  UpperLimitBound=pi/2  UpperLimitBoundUnits=rad  UpperLimitStiffness=0  UpperLimitStiffnessUnits=N*m/deg  UpperLimitDamping=0  UpperLimitDampingUnits=N*m/(deg/s)  UpperLimitTransitionRegionWidth=0.1  UpperLimitTransitionRegionWidthUnits=deg  PositionTargetSpecify=on  PositionTargetPriority=High  PositionTargetValue=q0(4)  PositionTargetValueUnits=rad  VelocityTargetSpecify=on  VelocityTargetPriority=High  VelocityTargetValue=dq0(4)  VelocityTargetValueUnits=rad/s
  joint_5 : sm_lib/Joints/Revolute Joint  JointMode=Normal  SenseConstraintForce=off  SenseConstraintForceX=off  SenseConstraintForceY=off  SenseConstraintForceZ=off  SenseConstraintTorque=off  SenseConstraintTorqueX=off  SenseConstraintTorqueY=off  SenseConstraintTorqueZ=off  SenseTotalForce=off  SenseTotalForceX=off  SenseTotalForceY=off  SenseTotalForceZ=off  SenseTotalTorque=off  SenseTotalTorqueX=off  SenseTotalTorqueY=off  SenseTotalTorqueZ=off  CompositeWrenchDir=FollowerOnBase  CompositeWrenchFrame=BaseFrame  EquilibriumPosition=0  EquilibriumPositionUnits=deg  SpringStiffness=0  SpringStiffnessUnits=N*m/deg  DampingCoefficient=0  DampingCoefficientUnits=kg*m^2/(rad*s)  TorqueActuationMode=InputTorque  MotionActuationMode=ComputedMotion  SensePosition=on  SenseVelocity=on  SenseAcceleration=on  SenseTorqueForce=on  SenseLowerLimitTorqueForce=off  SenseUpperLimitTorqueForce=off  LowerLimitSpecify=off  LowerLimitBound=-pi/2  LowerLimitBoundUnits=rad  LowerLimitStiffness=0  LowerLimitStiffnessUnits=N*m/deg  LowerLimitDamping=0  LowerLimitDampingUnits=N*m/(deg/s)  LowerLimitTransitionRegionWidth=0.1  LowerLimitTransitionRegionWidthUnits=deg  UpperLimitSpecify=off  UpperLimitBound=pi/2  UpperLimitBoundUnits=rad  UpperLimitStiffness=0  UpperLimitStiffnessUnits=N*m/deg  UpperLimitDamping=0  UpperLimitDampingUnits=N*m/(deg/s)  UpperLimitTransitionRegionWidth=0.1  UpperLimitTransitionRegionWidthUnits=deg  PositionTargetSpecify=on  PositionTargetPriority=High  PositionTargetValue=q0(5)  PositionTargetValueUnits=rad  VelocityTargetSpecify=on  VelocityTargetPriority=High  VelocityTargetValue=dq0(5)  VelocityTargetValueUnits=rad/s
  omuz : Subsystem
  on_kol : Subsystem
  tau_Demux : Demux  Outputs=5
  temasNoktasi : sm_lib/Frames and Transforms/Rigid Transform  TranslationMethod=Cartesian  TranslationStandardOffset=0  TranslationStandardOffsetUnits=m  TranslationStandardAxis=+Z  TranslationCartesianOffset=[0.0, 0, 0]  TranslationCartesianOffsetUnits=m  TranslationROffset=0  TranslationROffsetUnits=m  TranslationZOffset=0  TranslationZOffsetUnits=m  TranslationThetaOffset=0  TranslationThetaOffsetUnits=deg  RotationMethod=RotationSequence  RotationAngleUnits=deg  RotationStandardAxis=+Z  RotationAngle=0.0  RotationArbitraryAxis=[0 0 1]  FollAlignAxisA=+X  BaseAlignAxisA=+Y  FollAlignAxisB=+Y  BaseAlignAxisB=+Z  RotationSequenceAxes=BaseAxes  RotationSequence=XYZ  RotationSequenceAngles=[0, 0, 0]  RotationSequenceAnglesUnits=rad  RotationMatrix=[1 0 0; 0 1 0; 0 0 1]  Quaternion=[1 0 0 0]
  temel : Subsystem
  Uc Nokta : PMIOPort  Side=Left
  Referans : PMIOPort  Port=2  Side=Right
  Q_out : Outport
  Qdot_out : Outport  Port=2
  Qddot_out : Outport  Port=3
  Torq_out : Outport  Port=4
  wires:
  [Qddot_joint_2] -> Qdot_State Mux1/2
  [torq_joint_3] -> Qdot_State Mux2/3
  [Q_joint_4] -> Q_State Mux/4
  [Qdot_joint_3] -> Qdot_State Mux/3
  [Q_joint_5] -> Q_State Mux/5
  [Qdot_joint_5] -> Qdot_State Mux/5
  [torq_joint_5] -> Qdot_State Mux2/5
  [Qddot_joint_1] -> Qdot_State Mux1/1
  reaction torque/1 -> Sum/2, Gain/1
  [Qdot_joint_1] -> Qdot_State Mux/1
  Sum/1 -> Torq_out/1
  [Q_joint_3] -> Q_State Mux/3
  tau_Demux/2 -> [tau_joint_2]
  [Qdot_joint_4] -> Qdot_State Mux/4
  [Q_joint_1] -> Q_State Mux/1
  [Q_joint_2] -> Q_State Mux/2
  [Qddot_joint_5] -> Qdot_State Mux1/5
  Gain/1 -> Scope1/1, Sum1/2
  [torq_joint_4] -> Qdot_State Mux2/4
  tau_Demux/5 -> [tau_joint_5]
  [Qddot_joint_4] -> Qdot_State Mux1/4
  Sum1/1 -> tau_Demux/1
  Qdot_State Mux2/1 -> Sum/1
  tau_in/1 -> Sum1/1
  [torq_joint_1] -> Qdot_State Mux2/1
  Qdot_State Mux/1 -> Qdot_out/1
  Qdot_State Mux1/1 -> Qddot_out/1
  tau_Demux/3 -> [tau_joint_3]
  tau_Demux/4 -> [tau_joint_4]
  [Qdot_joint_2] -> Qdot_State Mux/2
  [torq_joint_2] -> Qdot_State Mux2/2
  Q_State Mux/1 -> Q_out/1
  [Qddot_joint_3] -> Qdot_State Mux1/3
  tau_Demux/1 -> [tau_joint_1]
  PSS Q_shoulder_pan_joint/1 -> [Q_joint_1]
  PSS Qddot_shoulder_pan_joint1/1 -> [torq_joint_1]
  PSS Qddot_shoulder_pan_joint/1 -> [Qddot_joint_1]
  PSS Qdot_shoulder_pan_joint/1 -> [Qdot_joint_1]
  PSS Qdot_shoulder_lift_joint/1 -> [Qdot_joint_2]
  PSS Qddot_shoulder_lift_joint/1 -> [Qddot_joint_2]
  PSS Q_shoulder_lift_joint/1 -> [Q_joint_2]
  PSS Qddot_shoulder_pan_joint2/1 -> [torq_joint_2]
  PSS Qddot_elbow_joint/1 -> [Qddot_joint_3]
  PSS Qddot_shoulder_pan_joint3/1 -> [torq_joint_3]
  PSS Q_elbow_joint/1 -> [Q_joint_3]
  PSS Qdot_elbow_joint/1 -> [Qdot_joint_3]
  PSS Q_wrist_1_joint/1 -> [Q_joint_4]
  PSS Qdot_wrist_1_joint/1 -> [Qdot_joint_4]
  PSS Qddot_shoulder_pan_joint4/1 -> [torq_joint_4]
  PSS Qddot_wrist_1_joint/1 -> [Qddot_joint_4]
  PSS Q_wrist_2_joint/1 -> [Q_joint_5]
  PSS Qdot_wrist_2_joint/1 -> [Qdot_joint_5]
  PSS Qddot_wrist_2_joint/1 -> [Qddot_joint_5]
  PSS Qddot_shoulder_pan_joint5/1 -> [torq_joint_5]
  [tau_joint_1] -> SPS tau_shoulder_pan_joint/1
  [tau_joint_2] -> SPS tau_shoulder_lift_joint/1
  [tau_joint_3] -> SPS tau_elbow_joint/1
  [tau_joint_4] -> SPS tau_wrist_1_joint/1
  [tau_joint_5] -> SPS tau_wrist_2_joint/1
  connections:
  MechanismConfiguration/RConn1 -- World/RConn1 -- temel/LConn1 -- Referans/RConn1 -- Solver Configuration/RConn1
  omuz/RConn1 -- joint_2/LConn1
  joint_4/RConn5 -- PSS Qddot_shoulder_pan_joint4/LConn1
  joint_5/RConn2 -- PSS Q_wrist_2_joint/LConn1
  joint_4/LConn1 -- dirsek/RConn1
  arka_kol/LConn1 -- joint_2/RConn1
  el_ve_bilek1/LConn1 -- joint_5/RConn1
  temel/RConn1 -- joint_1/LConn1
  omuz/LConn1 -- joint_1/RConn1
  on_kol/LConn1 -- joint_4/RConn1
  GripperLink/RConn1 -- Spherical Solid/RConn1 -- temasNoktasi/LConn1
  joint_4/RConn2 -- PSS Q_wrist_1_joint/LConn1
  joint_3/RConn2 -- PSS Q_elbow_joint/LConn1
  el_ve_bilek1/RConn1 -- GripperLink/LConn1
  joint_5/RConn5 -- PSS Qddot_shoulder_pan_joint5/LConn1
  PSS Qddot_shoulder_pan_joint/LConn1 -- joint_1/RConn4
  dirsek/LConn1 -- joint_3/RConn1
  on_kol/RConn1 -- joint_5/LConn1
  joint_3/LConn1 -- arka_kol/RConn1
  joint_5/RConn4 -- PSS Qddot_wrist_2_joint/LConn1
  joint_4/RConn4 -- PSS Qddot_wrist_1_joint/LConn1
  joint_4/RConn3 -- PSS Qdot_wrist_1_joint/LConn1
  joint_5/RConn3 -- PSS Qdot_wrist_2_joint/LConn1
  joint_3/RConn5 -- PSS Qddot_shoulder_pan_joint3/LConn1
  SPS tau_wrist_1_joint/RConn1 -- joint_4/LConn2
  SPS tau_elbow_joint/RConn1 -- joint_3/LConn2
  SPS tau_shoulder_lift_joint/RConn1 -- joint_2/LConn2
  SPS tau_shoulder_pan_joint/RConn1 -- joint_1/LConn2
  joint_1/RConn2 -- PSS Q_shoulder_pan_joint/LConn1
  joint_1/RConn3 -- PSS Qdot_shoulder_pan_joint/LConn1
  joint_1/RConn5 -- PSS Qddot_shoulder_pan_joint1/LConn1
  joint_2/RConn2 -- PSS Q_shoulder_lift_joint/LConn1
  joint_2/RConn3 -- PSS Qdot_shoulder_lift_joint/LConn1
  joint_2/RConn5 -- PSS Qddot_shoulder_pan_joint2/LConn1
  joint_2/RConn4 -- PSS Qddot_shoulder_lift_joint/LConn1
  joint_3/RConn4 -- PSS Qddot_elbow_joint/LConn1
  joint_3/RConn3 -- PSS Qdot_elbow_joint/LConn1
  joint_5/LConn2 -- SPS tau_wrist_2_joint/RConn1
  temasNoktasi/RConn1 -- Uc Nokta/RConn1
